simulink model "SimulinkOQPSK"  (R2024b)
settings: Solver=VariableStepAuto  StartTime=0.0  StopTime=10e-3  RelTol=1e-3
libraries: commutil2 x4, dspstat3 x4, commdigbbndpm3 x3, commseqgen3 x2, commsync2 x2, commfilt2 x2, commchan3 x1, commrfcorlib x1, commsink2 x1, commrflib2 x1, commrandsrc3 x1
settings Model: Creator=skaug  LastModifiedBy=skaug

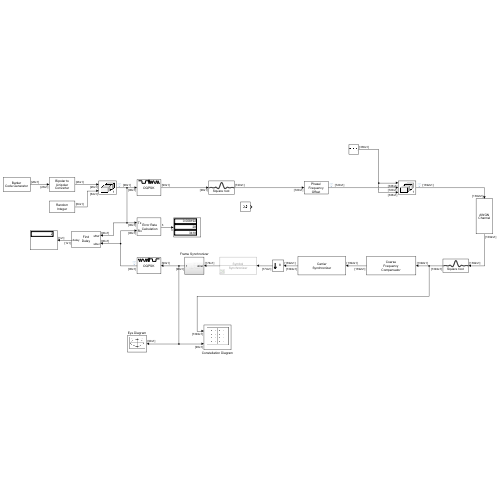
[thumbnail: Simulink's stored preview of the top-level diagram]
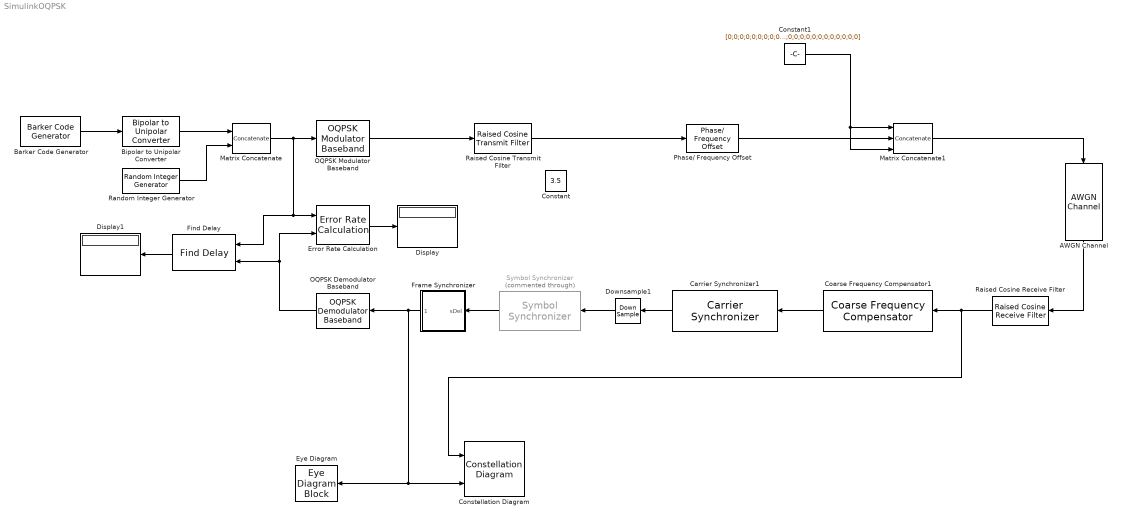
== system SimulinkOQPSK ==
  AWGN Channel : commchan3/AWGN Channel  LegacyMode=off  NoiseMethod="Signal to noise ratio  (Eb/No)"  noiseMode="Signal to noise ratio  (SNR)"  EbNo=20  EsNo=10  SNR=10  BitsPerSymbol=2  SignalPower=1  SamplesPerSymbol=8  SymbolPeriod=1  VarianceSource=Parameter  Variance=1  RandomStream=Global stream  Seed=67  SimulateUsing=Code generation
  Barker Code Generator : commseqgen3/Barker Code Generator  Length=7  LengthSimulink=13  SampleTime=-1  SamplesPerFrame=26  OutputDataType=double  SimulateUsing=Code generation
  Bipolar to Unipolar Converter : commutil2/Bipolar to Unipolar Converter  M=2  polarity=Positive  dataType=Inherit via internal rule
  Carrier Synchronizer1 : commsync2/Carrier Synchronizer  Modulation=OQPSK  ModulationPhaseOffset=Auto  CustomPhaseOffset=pi/4  SamplesPerSymbol=8  DampingFactor=0.707  NormalizedLoopBandwidth=0.01  EstimatedPhaseErrorOutputPort=off  SimulateUsing=Code generation
  Coarse Frequency Compensator1 : commrfcorlib/Coarse Frequency Compensator  Modulation=OQPSK  Algorithm=FFT-based  FrequencyResolution=100  MaximumFrequencyOffset=5e3  SamplesPerSymbol=8  EstimatedFreqOffsetPort=off  SimulateUsing=Code generation
      settings: LibrarySourceBlock=|
      | commsync2/Coarse Frequency
      | Compensator
  Constant : Constant  Value=3.5  SampleTime=1e-5
  Constant1 : Constant  Value=[0;0;0;0;0;0;0;0;0;0;0;0;0;0;0;0;0;0;0;0;0;0;0;0;0;0;0;0;0;0;0;0;0;0;0;0;0;0;0;0;0;0;0;0;0;0;0;0;0;0;0;0;0;0;0;0;0;0;0;0;0;0;0;0;0;0;0;0;0;0;0;0;0;0;0;0;0;0;0;0;0;0;0;0;0;0;0;0;0;0;0;0;0;0;0;0;0;0;0;0;0;0;0;0;0;0;0;0;0;0;0;0;0;0;0;0;0;0;0;0;0;0;0;0;0;0;0;0;0;0;0;0;0;0;0;0;0;0;0;0;0;0;0;0;0;0;0;0;0;0;0;0;0;0;0;0;0;0;0;0;0;0;0;0;0;0;0;0;0;0;0;0;0;0;0;0;0;0;0;0;0;0;0;0;0;0;0;0;0;0;0;0;0;0;0;0;0;0;0;0;0;0;0;0;0;0;0;0;0;0;0;0;0;0;0;0;0;0;0;0;0;0;0;0;0;0;0;0;0;0;0;0;0;0;0;0;0;0;0;0;0;0;0;0;0;0;0;0;0;0;0;0;0;0;0;0;0;0;0;0;0;0;0;0;0;0;0;0;0;0;0;0;0;0;0;0;0;0;0;0;0;0;0;0;0;0;0;0;0;0;0;0;0;0;0;0;0;0;0;0;0;0;0;0;0;0;0;0;0;0;0;0;0;0;0;0;0;0;0;0;0;0;0;0;0;0;0;0;0;0;0;0;0;0;0;0]  VectorParams1D=off  SampleTime=-1
  Constellation Diagram : ConstellationDiagram  NumInputPorts=2  WindowPosition=[306.000000,28.000000,801.000000,649.000000,]  ScopeFrameLocation=window  ReferenceConstellation="{[0.7071+0.7071i          -0.7071+0.7071i          -0.7071-0.7071i            0.707-0.7071i][0.7071+0.7071i          -0.7071+0.7071i          -0.7071-0.7071i            0.707-0.7071i]}"  ShowLegend=on
  Display : Display
  Display1 : Display
  Downsample1 : DownSample  N=8
  Error Rate Calculation : commsink2/Error Rate Calculation  N=2  st_delay=0  cp_mode=Entire frame  subframe=[]  PMode=Port  WsName=ErrorVec  RsMode2=off  stop=off  numErr=100  maxBits=1e6
  Eye Diagram : EyeDiagramBlock  WindowPosition=[70.000000,61.000000,1059.000000,721.000000,]  ScopeFrameLocation=window  SamplesPerSymbol=2  YLimits=[-1.1356977182574655,1.1330347719701188]  ColorFading=on
  Find Delay : commutil2/Find Delay  corrLength=200  chgSigOP=off  stopUpdate=off  numConstDelay=3
  Frame Synchronizer : Subsystem
  Matrix Concatenate : Concatenate  Mode=Multidimensional array
  Matrix Concatenate1 : Concatenate  NumInputs=3  Mode=Multidimensional array
  OQPSK Demodulator Baseband : commdigbbndpm3/OQPSK Demodulator Baseband  OutType=Bit  Ph=pi/4  Mapping=Gray  pulseShape=Half sine  num=[0.7071, 0.7071]  rolloff=0.2  filterSpan=10  sps=2  RateOptions=Enforce single-rate processing  outDtype2=double
  OQPSK Modulator Baseband : commdigbbndpm3/OQPSK Modulator Baseband  VariantControl=strcmp(pulseShape, 'Custom') && isequal(denom, 1)  InType=Bit  Mapping=Gray  Ph=pi/4  pulseShape=Half sine  num=[0.7071, 0.7071]  denom=[1]  rolloff=0.2  filterSpan=10  sps=2  RateOptions=Enforce single-rate processing  outDtype=double  isIIR=off
  Phase/ Frequency Offset : commrflib2/Phase// Frequency Offset  phaseOffset=47  freqPort=off  freqOffset=6e4
  Raised Cosine Receive Filter : commfilt2/Raised Cosine Receive Filter  filtType=Square root  R=0.35  filtSpan=4  N=8  downFactor=1  downOffset=0  filterGain=1  InputProcessing=Columns as channels (frame based)  RateOptions=Enforce single-rate processing  framing=Mute  checkCoeff=off  variableName=rcRxFilt  currentFiltSpan=10  D=5  inputOffset=0  sampMode=Mute  saveAsFlag=0  rateMode=Downsampling  checkGain=Normalized  launchFVT=on  roundingMode=Floor  overflowMode=off  coeffDataTypeStr=Inherit: Same word length as input  coeffMin=[]  coeffMax=[]  coeffLastDataTypeStr=Inherit: Same word length as input  accumDataTypeStr=Inherit: Same as product output  accumLastDataTypeStr=Inherit: Same as product output  outputDataTypeStr=Inherit: Same as accumulator  outputMin=[]  outputMax=[]  outputLastDataTypeStr=Inherit: Same as accumulator
  Raised Cosine Transmit Filter : commfilt2/Raised Cosine Transmit Filter  filtType=Square root  R=0.35  filtSpan=4  N=8  filterGain=1  InputProcessing=Columns as channels (frame based)  RateOptions=Enforce single-rate processing  framing=Mute  checkCoeff=off  variableName=rcTxFilt  checkGain=Normalized  sampMode=Mute  saveAsFlag=0  currentFiltSpan=10  D=(10)/2  launchFVT=on  roundingMode=Floor  overflowMode=off  coeffDataTypeStr=Inherit: Same word length as input  coeffMin=[]  coeffMax=[]  coeffLastDataTypeStr=Inherit: Same word length as input  outputDataTypeStr=Inherit: Same as accumulator  outputMin=[]  outputMax=[]  outputLastDataTypeStr=Inherit: Same as accumulator
  Random Integer Generator : commrandsrc3/Random Integer Generator  SetSize=2  SeedSource=Auto  Seed=0  SampleTime=-1  SamplesPerFrame=64  OutputDataType=double  SimulateUsing=Code generation
  Symbol Synchronizer : commsync2/Symbol Synchronizer  Commented=through  Modulation=OQPSK  TimingErrorDetector=Gardner (non-data-aided)  SamplesPerSymbol=8  DampingFactor=1  NormalizedLoopBandwidth=0.01  DetectorGain=2.7  TimingErrorOutputPort=off  SimulateUsing=Code generation
  wires:
  Barker Code Generator/1 -> Bipolar to Unipolar Converter/1
  OQPSK Modulator Baseband/1 -> Raised Cosine Transmit Filter/1
  Error Rate Calculation/1 -> Display/1
  OQPSK Demodulator Baseband/1 -> Error Rate Calculation/2, Find Delay/2
  Raised Cosine Receive Filter/1 -> Coarse Frequency Compensator1/1, Constellation Diagram/1
  Carrier Synchronizer1/1 -> Downsample1/1
  Coarse Frequency Compensator1/1 -> Carrier Synchronizer1/1
  Bipolar to Unipolar Converter/1 -> Matrix Concatenate/1
  Random Integer Generator/1 -> Matrix Concatenate/2
  Frame Synchronizer/1(Output) -> OQPSK Demodulator Baseband/1, Constellation Diagram/2, Eye Diagram/1
  AWGN Channel/1 -> Raised Cosine Receive Filter/1
  Phase/ Frequency Offset/1 -> Matrix Concatenate1/2
  Matrix Concatenate1/1 -> AWGN Channel/1
  Matrix Concatenate/1 -> Find Delay/1, Error Rate Calculation/1, OQPSK Modulator Baseband/1
  Constant1/1 -> Matrix Concatenate1/3, Matrix Concatenate1/1
  Find Delay/1 -> Display1/1
  Raised Cosine Transmit Filter/1 -> Phase/ Frequency Offset/1
  Downsample1/1 -> Symbol Synchronizer/1
  Symbol Synchronizer/1 -> Frame Synchronizer/1(sDel)

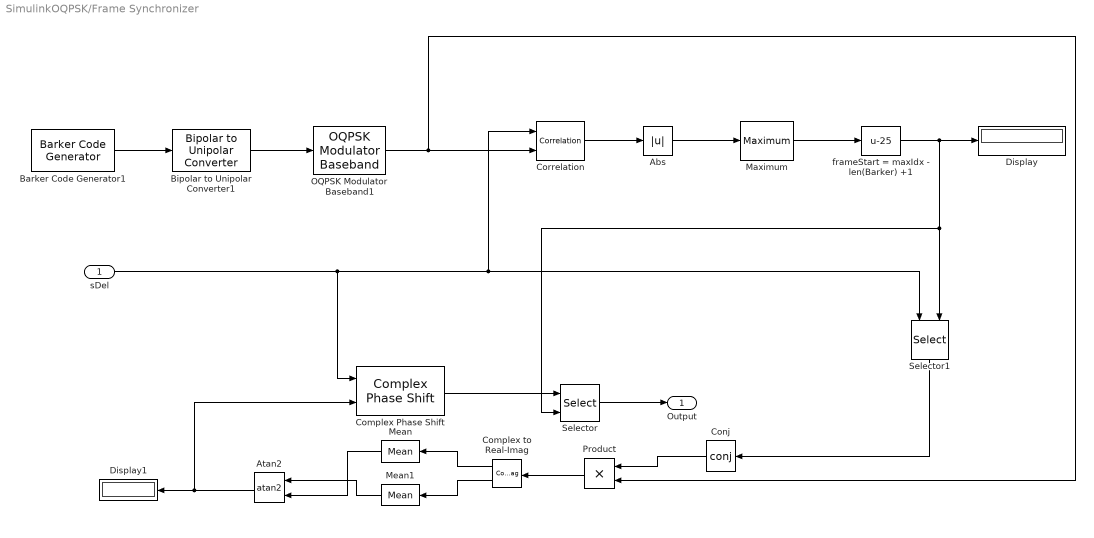
== system SimulinkOQPSK/Frame Synchronizer ==
  sDel : Inport
  Abs : Abs  SaturateOnIntegerOverflow=off
  Atan2 : Trigonometry  Operator=atan2
  Barker Code Generator1 : commseqgen3/Barker Code Generator  Length=7  LengthSimulink=13  SampleTime=-1  SamplesPerFrame=26  OutputDataType=double  SimulateUsing=Code generation
  Bipolar to Unipolar Converter1 : commutil2/Bipolar to Unipolar Converter  M=2  polarity=Positive  dataType=Inherit via internal rule
  Complex Phase Shift : commutil2/Complex Phase Shift
  Complex to Real-Imag : ComplexToRealImag
  Conj : Math  Operator=conj
  Correlation : dspstat3/Correlation  domain=Time  roundingMode=Floor  overflowMode=off  outputDataTypeStr=Inherit: Same as accumulator  outputMin=[]  outputMax=[]  outputLastDataTypeStr=Inherit: Same as accumulator
  Display : Display
  Display1 : Display
  Maximum : dspstat3/Maximum  operation=maximum  fcn=Index  indexBase=One  operateOver=Each column  Dimension=1  InputProcessing=Columns as channels (frame based)  reset=None  roiEnable=off  roiType=Rectangles  roiPortion=Entire ROI  roiOutput=Individual statistics for each ROI  roiFlag=off  roundingMode=Floor  overflowMode=off  accumDataTypeStr=Inherit: Same as product output  accumLastDataTypeStr=Inherit: Same as product output
  Mean : dspstat3/Mean  run=off  InputProcessing=Columns as channels (frame based)  reset_popup=None  directionMode=Each column  dimension=1  roiEnable=off  roiType=Rectangles  roiPortion=Entire ROI  roiOutput=Individual statistics for each ROI  roiFlag=off  roundingMode=Floor  overflowMode=off  outputDataTypeStr=Inherit: Same as accumulator  outputMin=[]  outputMax=[]  outputLastDataTypeStr=Inherit: Same as accumulator
  Mean1 : dspstat3/Mean  run=off  InputProcessing=Columns as channels (frame based)  reset_popup=None  directionMode=Each column  dimension=1  roiEnable=off  roiType=Rectangles  roiPortion=Entire ROI  roiOutput=Individual statistics for each ROI  roiFlag=off  roundingMode=Floor  overflowMode=off  outputDataTypeStr=Inherit: Same as accumulator  outputMin=[]  outputMax=[]  outputLastDataTypeStr=Inherit: Same as accumulator
  OQPSK Modulator Baseband1 : commdigbbndpm3/OQPSK Modulator Baseband  VariantControl=strcmp(pulseShape, 'Custom') && isequal(denom, 1)  InType=Bit  Mapping=Gray  Ph=pi/4  pulseShape=Half sine  num=[0.7071, 0.7071]  denom=[1]  rolloff=0.2  filterSpan=10  sps=2  RateOptions=Enforce single-rate processing  outDtype=double  isIIR=off
  Product : Product
  Selector : Selector  IndexOptions=Starting index (port)  Indices=[1 3]  OutputSizes=90
  Selector1 : Selector  IndexOptions=Starting index (port)  Indices=[1 3]  OutputSizes=26
  frameStart = maxIdx - len(Barker) +1 : Bias  Bias=-25  SaturateOnIntegerOverflow=off
  Output : Outport
  wires:
  sDel/1 -> Correlation/1, Selector1/1, Complex Phase Shift/1
  Complex to Real-Imag/2 -> Mean1/1
  Atan2/1 -> Complex Phase Shift/2, Display1/1
  OQPSK Modulator Baseband1/1 -> Product/2, Correlation/2
  Product/1 -> Complex to Real-Imag/1
  Mean/1 -> Atan2/2
  Bipolar to Unipolar Converter1/1 -> OQPSK Modulator Baseband1/1
  Barker Code Generator1/1 -> Bipolar to Unipolar Converter1/1
  Conj/1 -> Product/1
  Mean1/1 -> Atan2/1
  Complex to Real-Imag/1 -> Mean/1
  Complex Phase Shift/1 -> Selector/1
  Selector/1 -> Output/1
  Selector1/1 -> Conj/1
  Correlation/1 -> Abs/1
  Abs/1 -> Maximum/1
  frameStart = maxIdx - len(Barker) +1/1 -> Display/1, Selector/2, Selector1/2
  Maximum/1 -> frameStart = maxIdx - len(Barker) +1/1
